simulink model "triplex_12B_with_contracts_PP"  (R2019b)
settings: Solver=FixedStepDiscrete  StartTime=0.0  StopTime=10.0  FixedStep=0.100000  RelTol=1e-3  EnableMultiTasking=on
model workspace (MAT data in the model file):
  ContractValidatorBlocksMap : containers.Map (value not decoded)
  already_pp = 1
  compositionalMap : object (value not decoded)
  maskControlsMap : containers.Map (value not decoded)
  nodeNameToBlockNameMap : containers.Map (value not decoded)
  verificationResults : object (value not decoded)
undefined symbols (not defined in the file): contractAfterSimulation, contractBeforeSimulation, ContractBlock, ContractGuaranteeBlock, ContractValidatorBlock, saveValidatorParameters
(part 2 of 2)

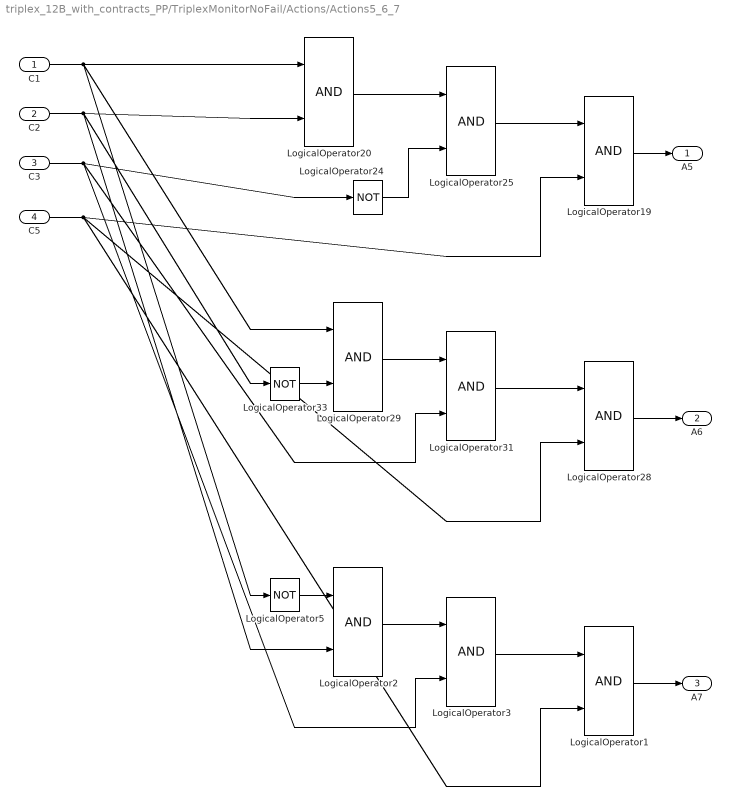
== system triplex_12B_with_contracts_PP/TriplexMonitorNoFail/Actions/Actions5_6_7 ==
  C1 : Inport
  C2 : Inport  Port=2
  C3 : Inport  Port=3
  C5 : Inport  Port=4
  LogicalOperator{1..3,19..20,25,28..29,31} (9 alike) : Logic  AllPortsSameDT=off  OutDataTypeStr=boolean
  LogicalOperator24 : Logic  Operator=NOT  Inputs=1  AllPortsSameDT=off  OutDataTypeStr=boolean
  LogicalOperator33 : Logic  Operator=NOT  Inputs=1  AllPortsSameDT=off  OutDataTypeStr=boolean
  LogicalOperator5 : Logic  Operator=NOT  Inputs=1  AllPortsSameDT=off  OutDataTypeStr=boolean
  A5 : Outport  VectorParamsAs1DForOutWhenUnconnected=off
  A6 : Outport  Port=2  VectorParamsAs1DForOutWhenUnconnected=off
  A7 : Outport  Port=3  VectorParamsAs1DForOutWhenUnconnected=off
  wires:
  LogicalOperator31/1 -> LogicalOperator28/1
  LogicalOperator29/1 -> LogicalOperator31/1
  C3/1 -> LogicalOperator24/1, LogicalOperator31/2, LogicalOperator3/2
  C2/1 -> LogicalOperator20/2, LogicalOperator33/1, LogicalOperator2/2
  LogicalOperator20/1 -> LogicalOperator25/1
  C5/1 -> LogicalOperator19/2, LogicalOperator28/2, LogicalOperator1/2
  LogicalOperator33/1 -> LogicalOperator29/2
  LogicalOperator25/1 -> LogicalOperator19/1
  LogicalOperator24/1 -> LogicalOperator25/2
  LogicalOperator19/1 -> A5/1
  LogicalOperator28/1 -> A6/1
  LogicalOperator3/1 -> LogicalOperator1/1
  C1/1 -> LogicalOperator5/1, LogicalOperator20/1, LogicalOperator29/1
  LogicalOperator2/1 -> LogicalOperator3/1
  LogicalOperator1/1 -> A7/1
  LogicalOperator5/1 -> LogicalOperator2/1

== system triplex_12B_with_contracts_PP/TriplexMonitorNoFail/Output/No_minus_Fail ==
  note: // Action 1: no-fail state
  ia : Inport
  ib : Inport  Port=2
  ic : Inport  Port=3
  ActionPort : ActionPort  ActionPortLabel=if(u1==0.0)
  Avg3 : Subsystem  TreatAsAtomicUnit=on
  choose : Subsystem  TreatAsAtomicUnit=on
  choose1 : Subsystem  TreatAsAtomicUnit=on
  sel_val : Outport  VectorParamsAs1DForOutWhenUnconnected=off
  wires:
  ib/1 -> Avg3/2(i2), choose/3(i2)
  ia/1 -> choose/1(i1), Avg3/1(i1)
  Avg3/1(Avg) -> choose1/2(avg), choose/2(avg)
  choose/1(choice) -> choose1/1(i1)
  ic/1 -> choose1/3(i2), Avg3/3(i3)
  choose1/1(choice) -> sel_val/1

== system triplex_12B_with_contracts_PP/TriplexMonitorNoFail/Output/Single_minus_BranchA_minus_Fail ==
  note: // Action 4: Single-BranchA-Fail
  ib : Inport
  ic : Inport  Port=2
  ActionPort : ActionPort  ActionPortLabel=elseif( u1==4.0)
  Avg2 : Subsystem  TreatAsAtomicUnit=on
  sel_val : Outport  VectorParamsAs1DForOutWhenUnconnected=off
  wires:
  Avg2/1(Avg) -> sel_val/1
  ic/1 -> Avg2/2(i2)
  ib/1 -> Avg2/1(i1)

== system triplex_12B_with_contracts_PP/TriplexMonitorNoFail/Output/Single_minus_BranchB_minus_Fail ==
  note: // Action 3: Single-BranchB-Fail
  ia : Inport
  ic : Inport  Port=2
  ActionPort : ActionPort  ActionPortLabel=elseif( u1==2.0)
  Avg2 : Subsystem  TreatAsAtomicUnit=on
  sel_val : Outport  VectorParamsAs1DForOutWhenUnconnected=off
  wires:
  ia/1 -> Avg2/1(i1)
  ic/1 -> Avg2/2(i2)
  Avg2/1(Avg) -> sel_val/1

== system triplex_12B_with_contracts_PP/TriplexMonitorNoFail/Output/Single_minus_BranchC_minus_Fail ==
  note: // Action 2: Single-BranchC-Fail
  ia : Inport
  ib : Inport  Port=2
  ActionPort : ActionPort  ActionPortLabel=elseif(u1==1.0)
  Avg2 : Subsystem  TreatAsAtomicUnit=on
  sel_val : Outport  VectorParamsAs1DForOutWhenUnconnected=off
  wires:
  Avg2/1(Avg) -> sel_val/1
  ib/1 -> Avg2/2(i2)
  ia/1 -> Avg2/1(i1)

== system triplex_12B_with_contracts_PP/TriplexMonitorNoFail/Output/No_minus_Fail/Avg3 ==
  i1 : Inport
  i2 : Inport  Port=2
  i3 : Inport  Port=3
  Constant : Constant  Value=3.0
  Divide : Product  Inputs=*/
  Sum : Sum  Inputs=|++
  Sum1 : Sum  Inputs=|++
  Avg : Outport  VectorParamsAs1DForOutWhenUnconnected=off
  wires:
  Sum1/1 -> Divide/1
  Constant/1 -> Divide/2
  i2/1 -> Sum/2
  Sum/1 -> Sum1/1
  Divide/1 -> Avg/1
  i3/1 -> Sum1/2
  i1/1 -> Sum/1

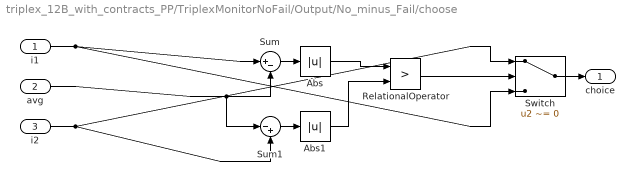
== system triplex_12B_with_contracts_PP/TriplexMonitorNoFail/Output/No_minus_Fail/choose ==
  i1 : Inport
  avg : Inport  Port=2
  i2 : Inport  Port=3
  Abs : Abs
  Abs1 : Abs
  RelationalOperator : RelationalOperator  Operator=>  OutDataTypeStr=boolean  RndMeth=Nearest
  Sum : Sum  Inputs=|+-
  Sum1 : Sum  Inputs=|-+
  Switch : Switch  Criteria=u2 ~= 0
  choice : Outport  VectorParamsAs1DForOutWhenUnconnected=off
  wires:
  Abs/1 -> RelationalOperator/1
  Switch/1 -> choice/1
  i1/1 -> Switch/3, Sum/1
  i2/1 -> Switch/1, Sum1/2
  Abs1/1 -> RelationalOperator/2
  Sum1/1 -> Abs1/1
  RelationalOperator/1 -> Switch/2
  Sum/1 -> Abs/1
  avg/1 -> Sum1/1, Sum/2

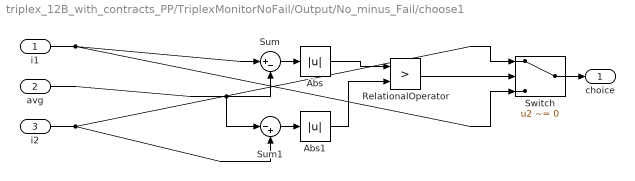
== system triplex_12B_with_contracts_PP/TriplexMonitorNoFail/Output/No_minus_Fail/choose1 ==
  i1 : Inport
  avg : Inport  Port=2
  i2 : Inport  Port=3
  Abs : Abs
  Abs1 : Abs
  RelationalOperator : RelationalOperator  Operator=>  OutDataTypeStr=boolean  RndMeth=Nearest
  Sum : Sum  Inputs=|+-
  Sum1 : Sum  Inputs=|-+
  Switch : Switch  Criteria=u2 ~= 0
  choice : Outport  VectorParamsAs1DForOutWhenUnconnected=off
  wires:
  avg/1 -> Sum/2, Sum1/1
  Sum/1 -> Abs/1
  RelationalOperator/1 -> Switch/2
  Sum1/1 -> Abs1/1
  Abs1/1 -> RelationalOperator/2
  i2/1 -> Switch/1, Sum1/2
  i1/1 -> Switch/3, Sum/1
  Switch/1 -> choice/1
  Abs/1 -> RelationalOperator/1

== system triplex_12B_with_contracts_PP/TriplexMonitorNoFail/Output/Single_minus_BranchA_minus_Fail/Avg2 ==
  i1 : Inport
  i2 : Inport  Port=2
  Constant : Constant  Value=2.0
  Divide : Product  Inputs=*/
  Sum : Sum  Inputs=|++
  Avg : Outport  VectorParamsAs1DForOutWhenUnconnected=off
  wires:
  i1/1 -> Sum/1
  Divide/1 -> Avg/1
  i2/1 -> Sum/2
  Constant/1 -> Divide/2
  Sum/1 -> Divide/1

== system triplex_12B_with_contracts_PP/TriplexMonitorNoFail/Output/Single_minus_BranchB_minus_Fail/Avg2 ==
  i1 : Inport
  i2 : Inport  Port=2
  Constant : Constant  Value=2.0
  Divide : Product  Inputs=*/
  Sum : Sum  Inputs=|++
  Avg : Outport  VectorParamsAs1DForOutWhenUnconnected=off
  wires:
  Sum/1 -> Divide/1
  Constant/1 -> Divide/2
  i2/1 -> Sum/2
  Divide/1 -> Avg/1
  i1/1 -> Sum/1

== system triplex_12B_with_contracts_PP/TriplexMonitorNoFail/Output/Single_minus_BranchC_minus_Fail/Avg2 ==
  i1 : Inport
  i2 : Inport  Port=2
  Constant : Constant  Value=2.0
  Divide : Product  Inputs=*/
  Sum : Sum  Inputs=|++
  Avg : Outport  VectorParamsAs1DForOutWhenUnconnected=off
  wires:
  i1/1 -> Sum/1
  Divide/1 -> Avg/1
  i2/1 -> Sum/2
  Constant/1 -> Divide/2
  Sum/1 -> Divide/1
